simulink model "data_integration"  (R2025b)
settings: Solver=VariableStepAuto  StartTime=0.0  StopTime=100  RelTol=1e-3
settings Model: Creator=jak64  LastModifiedBy=jak64

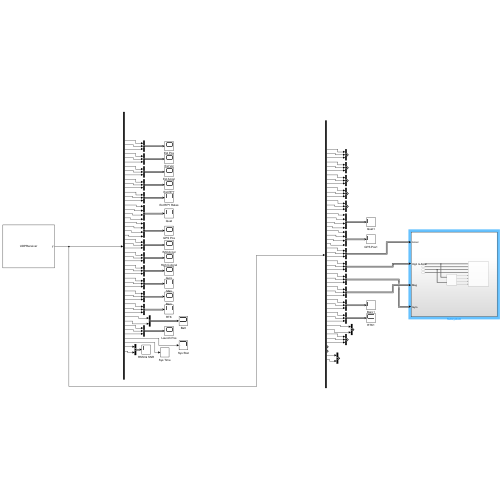
[thumbnail: Simulink's stored preview of the top-level diagram]
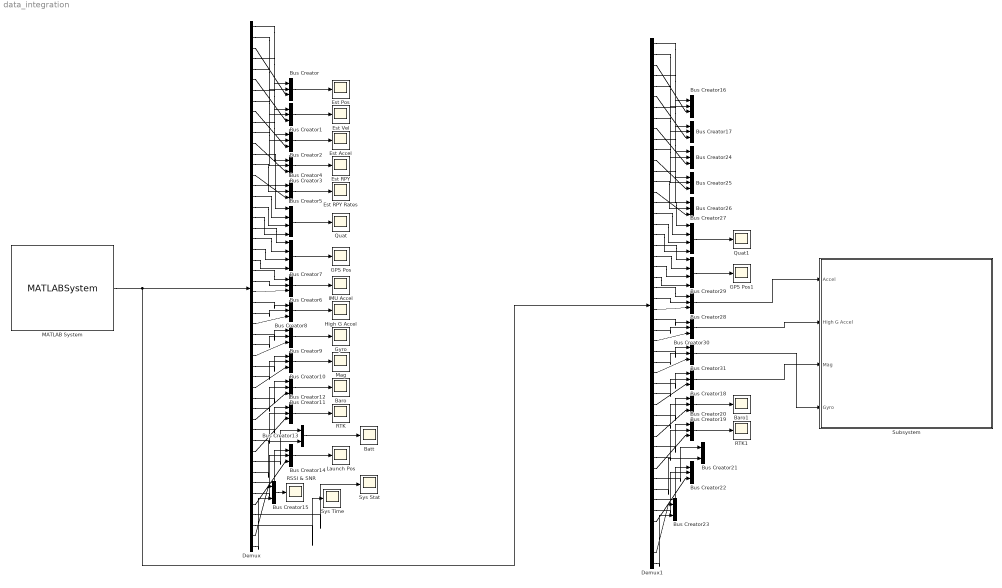
== system data_integration ==
  Baro : Scope
      settings: ActiveDisplayYMinimum=-1  ActiveDisplayYMaximum=1  DataLoggingVariableName=ScopeData6
  Baro1 : Scope
      settings: ActiveDisplayYMinimum=-1  ActiveDisplayYMaximum=1  DataLoggingVariableName=ScopeData18
  Batt : Scope
      settings: ActiveDisplayYMinimum=-1  ActiveDisplayYMaximum=1  DataLoggingVariableName=ScopeData8
  Bus Creator{,1..4,6,8..12,14,16..20,22,24..26,28,30..31} (24 alike) : BusCreator  Inputs=3
  Bus Creator{13,15,21,23} (4 alike) : BusCreator  Inputs=2
  Bus Creator{5,7,27,29} (4 alike) : BusCreator  Inputs=4
  Demux : Demux  Outputs=50
  Demux1 : Demux  Outputs=50
  Est Accel : Scope
      settings: ActiveDisplayYMinimum=-7.078610757242493  ActiveDisplayYMaximum=4.0316027838887836  DataLoggingVariableName=ScopeData10
  Est Pos : Scope
      settings: ActiveDisplayYMinimum=-7.078610757242493  ActiveDisplayYMaximum=4.0316027838887836  DataLoggingVariableName=ScopeData12
  Est RPY : Scope
      settings: ActiveDisplayYMinimum=-0.10932677163042247  ActiveDisplayYMaximum=0.034337563481739025
  Est RPY Rates : Scope
      settings: ActiveDisplayYMinimum=-0.410589762032032  ActiveDisplayYMaximum=0.64355004578828812  DataLoggingVariableName=ScopeData13
  Est Vel : Scope
      settings: ActiveDisplayYMinimum=-7.078610757242493  ActiveDisplayYMaximum=4.0316027838887836  DataLoggingVariableName=ScopeData11
  GPS Pos : Scope
      settings: ActiveDisplayYMinimum=-1  ActiveDisplayYMaximum=1  DataLoggingVariableName=ScopeData14
  GPS Pos1 : Scope
      settings: ActiveDisplayYMinimum=-1  ActiveDisplayYMaximum=1  DataLoggingVariableName=ScopeData25
  Gyro : Scope
      settings: ActiveDisplayYMinimum=-1  ActiveDisplayYMaximum=1  DataLoggingVariableName=ScopeData4
  High G Accel : Scope
      settings: ActiveDisplayYMinimum=-2.4089908003807068  ActiveDisplayYMaximum=0.67456668615341187
  IMU Accel : Scope
      settings: ActiveDisplayYMinimum=-1.354182630777359  ActiveDisplayYMaximum=1.1817843019962311  DataLoggingVariableName=ScopeData3
  Launch Pos : Scope
      settings: ActiveDisplayYMinimum=-1  ActiveDisplayYMaximum=1  DataLoggingVariableName=ScopeData9
  MATLAB System : MATLABSystem  System=UDPReceiver  port=5005
      mask Type: UDPReceiver
  Mag : Scope
      settings: ActiveDisplayYMinimum=-1  ActiveDisplayYMaximum=1  DataLoggingVariableName=ScopeData5
  Quat : Scope
      settings: ActiveDisplayYMinimum=-1.043480820953846  ActiveDisplayYMaximum=0.45715559273958206  DataLoggingVariableName=ScopeData2
  Quat1 : Scope
      settings: ActiveDisplayYMinimum=-1  ActiveDisplayYMaximum=1  DataLoggingVariableName=ScopeData31
  RSSI & SNR : Scope
      settings: ActiveDisplayYMinimum=-131.21875  ActiveDisplayYMaximum=0.96874999999999645  DataLoggingVariableName=ScopeData17
  RTK : Scope
      settings: ActiveDisplayYMinimum=-1  ActiveDisplayYMaximum=1  DataLoggingVariableName=ScopeData7
  RTK1 : Scope
      settings: ActiveDisplayYMinimum=-1  ActiveDisplayYMaximum=1  DataLoggingVariableName=ScopeData33
  Subsystem : Subsystem
  Sys Stat : Scope
      settings: ActiveDisplayYMinimum=-1  ActiveDisplayYMaximum=1  DataLoggingVariableName=ScopeData15
  Sys Time : Scope
      settings: ActiveDisplayYMinimum=-1  ActiveDisplayYMaximum=1  DataLoggingVariableName=ScopeData16
  wires:
  MATLAB System/1 -> Demux/1, Demux1/1
  Demux/1 -> Bus Creator/1
  Demux/2 -> Bus Creator/2
  Demux/3 -> Bus Creator/3
  Demux/5 -> Bus Creator1/2
  Demux/4 -> Bus Creator1/1
  Demux/6 -> Bus Creator1/3
  Demux/8 -> Bus Creator2/2
  Demux/7 -> Bus Creator2/1
  Demux/9 -> Bus Creator2/3
  Demux/11 -> Bus Creator3/2
  Demux/10 -> Bus Creator3/1
  Demux/12 -> Bus Creator3/3
  Bus Creator3/1 -> Est RPY/1
  Demux/13 -> Bus Creator4/1
  Demux/14 -> Bus Creator4/2
  Demux/15 -> Bus Creator4/3
  Demux/16 -> Bus Creator5/1
  Demux/17 -> Bus Creator5/2
  Demux/18 -> Bus Creator5/3
  Demux/19 -> Bus Creator5/4
  Bus Creator5/1 -> Quat/1
  Demux/20 -> Bus Creator7/1
  Demux/21 -> Bus Creator7/2
  Demux/22 -> Bus Creator7/3
  Demux/23 -> Bus Creator7/4
  Demux/25 -> Bus Creator6/2
  Demux/24 -> Bus Creator6/1
  Demux/26 -> Bus Creator6/3
  Bus Creator6/1 -> IMU Accel/1
  Demux/28 -> Bus Creator8/2
  Demux/27 -> Bus Creator8/1
  Demux/29 -> Bus Creator8/3
  Bus Creator8/1 -> High G Accel/1
  Demux/31 -> Bus Creator9/2
  Bus Creator9/1 -> Gyro/1
  Demux/32 -> Bus Creator9/3
  Demux/30 -> Bus Creator9/1
  Demux/34 -> Bus Creator10/2
  Bus Creator10/1 -> Mag/1
  Demux/35 -> Bus Creator10/3
  Demux/33 -> Bus Creator10/1
  Demux/37 -> Bus Creator11/2
  Bus Creator11/1 -> Baro/1
  Demux/38 -> Bus Creator11/3
  Demux/36 -> Bus Creator11/1
  Demux/40 -> Bus Creator12/2
  Bus Creator12/1 -> RTK/1
  Demux/41 -> Bus Creator12/3
  Demux/39 -> Bus Creator12/1
  Demux/43 -> Bus Creator13/2
  Bus Creator13/1 -> Batt/1
  Demux/42 -> Bus Creator13/1
  Demux/45 -> Bus Creator14/2
  Bus Creator14/1 -> Launch Pos/1
  Demux/46 -> Bus Creator14/3
  Demux/44 -> Bus Creator14/1
  Bus Creator7/1 -> GPS Pos/1
  Bus Creator/1 -> Est Pos/1
  Bus Creator1/1 -> Est Vel/1
  Bus Creator2/1 -> Est Accel/1
  Bus Creator4/1 -> Est RPY Rates/1
  Demux/47 -> Sys Stat/1
  Demux/48 -> Sys Time/1
  Demux/49 -> Bus Creator15/1
  Demux/50 -> Bus Creator15/2
  Bus Creator15/1 -> RSSI & SNR/1
  Demux1/14 -> Bus Creator26/2
  Demux1/7 -> Bus Creator24/1
  Demux1/10 -> Bus Creator25/1
  Demux1/4 -> Bus Creator17/1
  Demux1/12 -> Bus Creator25/3
  Demux1/43 -> Bus Creator21/2
  Demux1/42 -> Bus Creator21/1
  Demux1/44 -> Bus Creator22/1
  Demux1/46 -> Bus Creator22/3
  Demux1/11 -> Bus Creator25/2
  Bus Creator19/1 -> Baro1/1
  Demux1/28 -> Bus Creator30/2
  Demux1/38 -> Bus Creator19/3
  Demux1/32 -> Bus Creator31/3
  Demux1/45 -> Bus Creator22/2
  Demux1/31 -> Bus Creator31/2
  Demux1/33 -> Bus Creator18/1
  Demux1/16 -> Bus Creator27/1
  Demux1/24 -> Bus Creator28/1
  Demux1/23 -> Bus Creator29/4
  Demux1/1 -> Bus Creator16/1
  Demux1/21 -> Bus Creator29/2
  Demux1/36 -> Bus Creator19/1
  Bus Creator18/1 -> Subsystem/3(Mag)
  Bus Creator28/1 -> Subsystem/1(Accel)
  Demux1/8 -> Bus Creator24/2
  Demux1/3 -> Bus Creator16/3
  Bus Creator31/1 -> Subsystem/4(Gyro)
  Bus Creator30/1 -> Subsystem/2(High G Accel)
  Demux1/37 -> Bus Creator19/2
  Demux1/39 -> Bus Creator20/1
  Bus Creator27/1 -> Quat1/1
  Demux1/40 -> Bus Creator20/2
  Demux1/30 -> Bus Creator31/1
  Demux1/6 -> Bus Creator17/3
  Demux1/34 -> Bus Creator18/2
  Demux1/19 -> Bus Creator27/4
  Demux1/22 -> Bus Creator29/3
  Demux1/2 -> Bus Creator16/2
  Demux1/35 -> Bus Creator18/3
  Demux1/15 -> Bus Creator26/3
  Demux1/50 -> Bus Creator23/2
  Demux1/29 -> Bus Creator30/3
  Demux1/13 -> Bus Creator26/1
  Demux1/41 -> Bus Creator20/3
  Demux1/26 -> Bus Creator28/3
  Demux1/18 -> Bus Creator27/3
  Demux1/17 -> Bus Creator27/2
  Bus Creator29/1 -> GPS Pos1/1
  Demux1/27 -> Bus Creator30/1
  Bus Creator20/1 -> RTK1/1
  Demux1/25 -> Bus Creator28/2
  Demux1/5 -> Bus Creator17/2
  Demux1/20 -> Bus Creator29/1
  Demux1/49 -> Bus Creator23/1
  Demux1/9 -> Bus Creator24/3

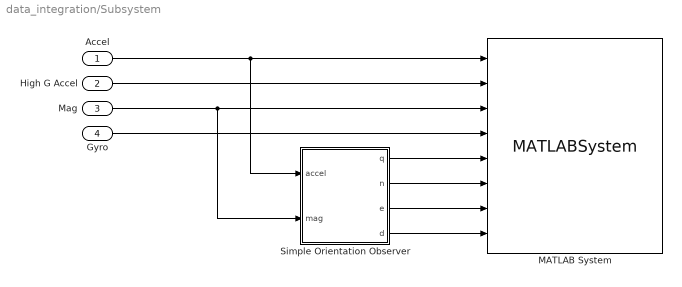
== system data_integration/Subsystem ==
  Accel : Inport
  High G Accel : Inport  Port=2
  Mag : Inport  Port=3
  Gyro : Inport  Port=4
  MATLAB System : MATLABSystem  System=Plotter
      mask Type: Plotter
  Simple Orientation Observer : MATLAB Function  TreatAsAtomicUnit=on
  wires:
  Accel/1 -> Simple Orientation Observer/1(accel), MATLAB System/1
  Gyro/1 -> MATLAB System/4
  Mag/1 -> Simple Orientation Observer/2(mag), MATLAB System/3
  High G Accel/1 -> MATLAB System/2
  Simple Orientation Observer/1(q) -> MATLAB System/5
  Simple Orientation Observer/4(d) -> MATLAB System/8
  Simple Orientation Observer/3(e) -> MATLAB System/7
  Simple Orientation Observer/2(n) -> MATLAB System/6

== matlab function data_integration/Subsystem/Simple Orientation Observer ==
  data: accel input; q output; mag input; n output; e output; d output
function [q, n, e, d]= fcn(accel, mag)
%#codegen

% --- Default outputs (safe values) ---
q = [1;0;0;0];
n = [1;0;0];
e = [0;1;0];
d = [0;0;1];

% Ensure column vectors
accel = accel(:);
mag   = mag(:);

% Normalize inputs (prevent NaN)
an = norm(accel);
mn = norm(mag);

if an < 1e-6 || mn < 1e-6
    return;   % ✅ all outputs already defined
end

accel = accel / an;
mag   = mag   / mn;

% Build orthonormal frame (NED style)
east  = cross(accel, mag);
en = norm(east);
if en < 1e-6
    return;   % ✅ all outputs already defined
end
east = east / en;

north = cross(east, accel);
north = north / norm(north);

down = accel; % already normalized

% Rotation matrix body->world
R = [north east down];

% Convert to quaternion
q = rotm2quat_custom(R);
n = north;
e = east;
d = down;
end


% -------------------------------------------------------
function q = rotm2quat_custom(R)
% Stable quaternion extraction for codegen

tr = R(1,1) + R(2,2) + R(3,3);

if tr > 0
    S = sqrt(tr + 1.0) * 2;
    qw = 0.25 * S;
    qx = (R(3,2) - R(2,3)) / S;
    qy = (R(1,3) - R(3,1)) / S;
    qz = (R(2,1) - R(1,2)) / S;

elseif (R(1,1) > R(2,2)) && (R(1,1) > R(3,3))
    S = sqrt(1.0 + R(1,1) - R(2,2) - R(3,3)) * 2;
    qw = (R(3,2) - R(2,3)) / S;
    qx = 0.25 * S;
    qy = (R(1,2) + R(2,1)) / S;
    qz = (R(1,3) + R(3,1)) / S;

elseif R(2,2) > R(3,3)
    S = sqrt(1.0 + R(2,2) - R(1,1) - R(3,3)) * 2;
    qw = (R(1,3) - R(3,1)) / S;
    qx = (R(1,2) + R(2,1)) / S;
    qy = 0.25 * S;
    qz = (R(2,3) + R(3,2)) / S;

else
    S = sqrt(1.0 + R(3,3) - R(1,1) - R(2,2)) * 2;
    qw = (R(2,1) - R(1,2)) / S;
    qx = (R(1,3) + R(3,1)) / S;
    qy = (R(2,3) + R(3,2)) / S;
    qz = 0.25 * S;
end

q = [qw; qx; qy; qz];

% Normalize
q = q / norm(q);
end
